simulink model "SingleAgent_Manipulator"  (R2018b)
settings: Solver=VariableStepAuto  StartTime=0.0  StopTime=10  RelTol=1e-3
values from neighbouring files (symbols this model uses):
  p02 = zeros(SInfo2.n, 1)    [Parameters.m]
  q01 = zeros(SInfo1.n, 1)    [Parameters.m]
settings Model: Creator=oscar  LastModifiedBy=oscar

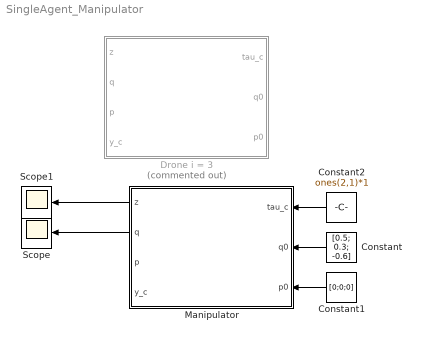
== system SingleAgent_Manipulator ==
  Constant : Constant  Value=[0.5; 0.3; -0.6]
  Constant1 : Constant  Value=[0;0;0]
  Constant2 : Constant  Value=ones(2,1)*1
  Drone i = 3 : Subsystem  Commented=on
  Manipulator : Subsystem
  Scope : Scope
  Scope1 : Scope
  wires:
  Constant/1 -> Manipulator/2(q0)
  Constant1/1 -> Manipulator/3(p0)
  Constant2/1 -> Manipulator/1(tau_c)
  Manipulator/2(q) -> Scope/1
  Manipulator/1(z) -> Scope1/1

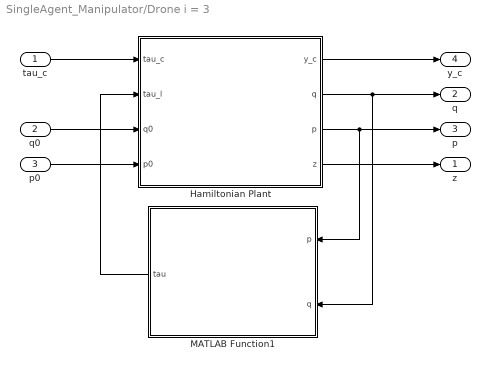
== system SingleAgent_Manipulator/Drone i = 3 ==
  tau_c : Inport
  q0 : Inport  Port=2
  p0 : Inport  Port=3
  Hamiltonian Plant : Subsystem
  MATLAB Function1 : MATLAB Function  TreatAsAtomicUnit=on
  z : Outport
  q : Outport  Port=2
  p : Outport  Port=3
  y_c : Outport  Port=4
  wires:
  MATLAB Function1/1(tau) -> Hamiltonian Plant/2(tau_l)
  tau_c/1 -> Hamiltonian Plant/1(tau_c)
  Hamiltonian Plant/3(p) -> MATLAB Function1/1(p), p/1
  Hamiltonian Plant/2(q) -> MATLAB Function1/2(q), q/1
  Hamiltonian Plant/4(z) -> z/1
  Hamiltonian Plant/1(y_c) -> y_c/1
  q0/1 -> Hamiltonian Plant/3(q0)
  p0/1 -> Hamiltonian Plant/4(p0)

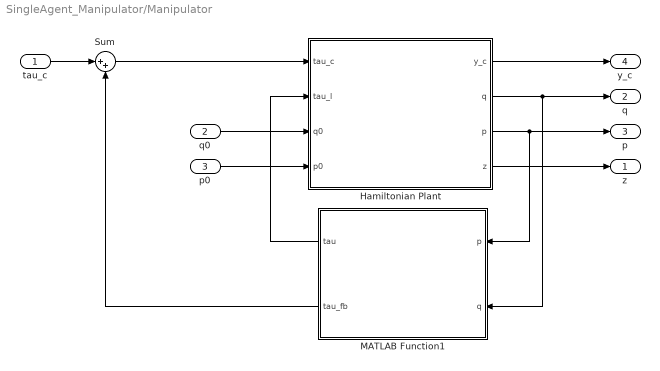
== system SingleAgent_Manipulator/Manipulator ==
  tau_c : Inport
  q0 : Inport  Port=2
  p0 : Inport  Port=3
  Hamiltonian Plant : Subsystem
  MATLAB Function1 : MATLAB Function  TreatAsAtomicUnit=on
  Sum : Sum  Inputs=|++
  z : Outport
  q : Outport  Port=2
  p : Outport  Port=3
  y_c : Outport  Port=4
  wires:
  MATLAB Function1/1(tau) -> Hamiltonian Plant/2(tau_l)
  tau_c/1 -> Sum/1
  Hamiltonian Plant/3(p) -> MATLAB Function1/1(p), p/1
  Hamiltonian Plant/2(q) -> MATLAB Function1/2(q), q/1
  Hamiltonian Plant/4(z) -> z/1
  Hamiltonian Plant/1(y_c) -> y_c/1
  q0/1 -> Hamiltonian Plant/3(q0)
  p0/1 -> Hamiltonian Plant/4(p0)
  MATLAB Function1/2(tau_fb) -> Sum/2
  Sum/1 -> Hamiltonian Plant/1(tau_c)

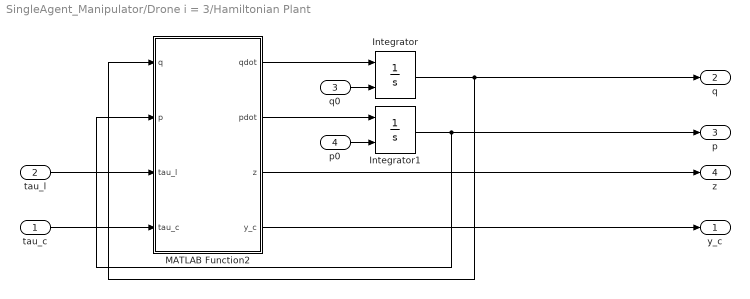
== system SingleAgent_Manipulator/Drone i = 3/Hamiltonian Plant ==
  tau_c : Inport
  tau_l : Inport  Port=2
  q0 : Inport  Port=3
  p0 : Inport  Port=4
  Integrator : Integrator  InitialConditionSource=external  InitialCondition=q01
  Integrator1 : Integrator  InitialConditionSource=external  InitialCondition=p02
  MATLAB Function2 : MATLAB Function  TreatAsAtomicUnit=on
  y_c : Outport
  q : Outport  Port=2
  p : Outport  Port=3
  z : Outport  Port=4
  wires:
  tau_l/1 -> MATLAB Function2/3(tau_l)
  MATLAB Function2/2(pdot) -> Integrator1/1
  Integrator1/1 -> MATLAB Function2/2(p), p/1
  Integrator/1 -> MATLAB Function2/1(q), q/1
  MATLAB Function2/1(qdot) -> Integrator/1
  p0/1 -> Integrator1/2
  MATLAB Function2/3(z) -> z/1
  tau_c/1 -> MATLAB Function2/4(tau_c)
  MATLAB Function2/4(y_c) -> y_c/1
  q0/1 -> Integrator/2

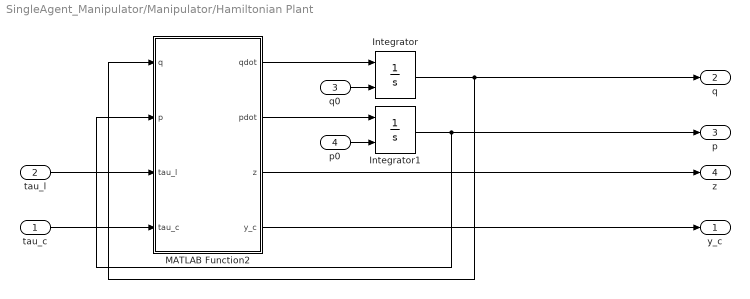
== system SingleAgent_Manipulator/Manipulator/Hamiltonian Plant ==
  tau_c : Inport
  tau_l : Inport  Port=2
  q0 : Inport  Port=3
  p0 : Inport  Port=4
  Integrator : Integrator  InitialConditionSource=external  InitialCondition=q01
  Integrator1 : Integrator  InitialConditionSource=external  InitialCondition=p02
  MATLAB Function2 : MATLAB Function  TreatAsAtomicUnit=on
  y_c : Outport
  q : Outport  Port=2
  p : Outport  Port=3
  z : Outport  Port=4
  wires:
  tau_l/1 -> MATLAB Function2/3(tau_l)
  MATLAB Function2/2(pdot) -> Integrator1/1
  Integrator1/1 -> MATLAB Function2/2(p), p/1
  Integrator/1 -> MATLAB Function2/1(q), q/1
  MATLAB Function2/1(qdot) -> Integrator/1
  p0/1 -> Integrator1/2
  MATLAB Function2/3(z) -> z/1
  tau_c/1 -> MATLAB Function2/4(tau_c)
  MATLAB Function2/4(y_c) -> y_c/1
  q0/1 -> Integrator/2

== matlab function SingleAgent_Manipulator/Drone i = 3/Hamiltonian Plant/MATLAB Function2 ==
  data: q input; qdot output; p input; tau_l input; pdot output; z output; tau_c input; y_c output
function [qdot, pdot, z, y_c] = fcn(q, p, tau_l, tau_c)

    coder.extrinsic('Drone1_Dynamics');
    qdot = zeros(3, 1);
    pdot = zeros(3, 1);
    z = zeros(2, 1);
    y_c = zeros(2, 1);
    [qdot, pdot, z, y_c] = Drone1_Dynamics(q, p, tau_l, tau_c);

== matlab function SingleAgent_Manipulator/Drone i = 3/MATLAB Function1 ==
  data: p input; q input; tau output
function tau = LocalControl(p, q)
    

coder.extrinsic('Drone1_Control');
tau = zeros(2, 1);
tau = Drone1_Control(q, p);

== matlab function SingleAgent_Manipulator/Manipulator/Hamiltonian Plant/MATLAB Function2 ==
  data: q input; qdot output; p input; tau_l input; pdot output; z output; tau_c input; y_c output
function [qdot, pdot, z, y_c] = fcn(q, p, tau_l, tau_c)

    coder.extrinsic('Manipulator_Dynamics');
    qdot = zeros(3, 1);
    pdot = zeros(3, 1);
    z = zeros(2, 1);
    y_c = zeros(2, 1);
    [qdot, pdot, z, y_c] = Manipulator_Dynamics(q, p, tau_l, tau_c);

== matlab function SingleAgent_Manipulator/Manipulator/MATLAB Function1 ==
  data: p input; q input; tau output; tau_fb output
function [tau, tau_fb] = LocalControl(p, q)
    

coder.extrinsic('Manipulator_Control');
tau = zeros(3, 1);
tau_fb = zeros(2, 1);
[tau, tau_fb] = Manipulator_Control(q, p);
